simulink model "sistema_controllato"  (R2019b)
settings: Solver=VariableStepAuto  StartTime=0.0  StopTime=10.0  RelTol=1e-3
undefined symbols (not defined in the file): den_G1, den_G2, den_Raa, den_Rd, den_Rpf, DENd, DENpf, mu, num_G1, num_G2, num_Raa, num_Rd, num_Rpf, NUMd, NUMpf, Ts
settings Model: Creator=edoardo  LastModifiedBy=edoardo

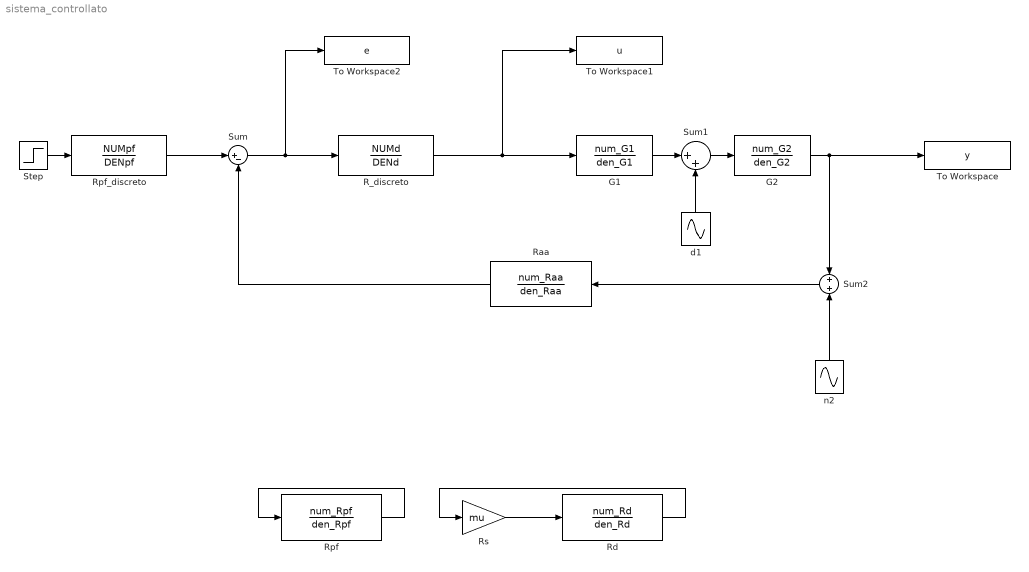
== system sistema_controllato ==
  "G1 " : TransferFcn  Numerator=num_G1  Denominator=den_G1
  G2 : TransferFcn  Numerator=num_G2  Denominator=den_G2
  "R_discreto " : DiscreteTransferFcn  Numerator=NUMd  Denominator=DENd  SampleTime=Ts
  Raa : TransferFcn  Numerator=num_Raa  Denominator=den_Raa
  Rd : TransferFcn  Numerator=num_Rd  Denominator=den_Rd
  Rpf : TransferFcn  Numerator=num_Rpf  Denominator=den_Rpf
  "Rpf_discreto " : DiscreteTransferFcn  Numerator=NUMpf  Denominator=DENpf  SampleTime=Ts
  Rs : Gain  Gain=mu
  Step : Step  Time=0  After=1.5  SampleTime=0
  Sum : Sum  Inputs=|+-
  Sum1 : Sum  Inputs=|++
  Sum2 : Sum
  To Workspace : ToWorkspace  VariableName=y  SaveFormat=Timeseries  SampleTime=-1
  To Workspace1 : ToWorkspace  VariableName=u  SaveFormat=Timeseries  SampleTime=-1
  To Workspace2 : ToWorkspace  VariableName=e  SaveFormat=Timeseries  SampleTime=-1
  d1 : Sin  Amplitude=3  SampleTime=0
  n2 : Sin  Amplitude=0.02  Frequency=8000  SampleTime=0
  wires:
  d1/1 -> Sum1/2
  "G1 "/1 -> Sum1/1
  Sum1/1 -> G2/1
  G2/1 -> Sum2/1, To Workspace/1
  Sum/1 -> "R_discreto "/1, To Workspace2/1
  n2/1 -> Sum2/2
  Sum2/1 -> Raa/1
  Raa/1 -> Sum/2
  Rs/1 -> Rd/1
  Rpf/1 -> Rpf/1
  Rd/1 -> Rs/1
  Step/1 -> "Rpf_discreto "/1
  "Rpf_discreto "/1 -> Sum/1
  "R_discreto "/1 -> To Workspace1/1, "G1 "/1
